simulink model "Tiefpass"  (R2023b)
settings: Solver=VariableStepAuto  StartTime=0.0  StopTime=1  RelTol=1e-3
settings Model: Creator=Adrian  LastModifiedBy=Adrian

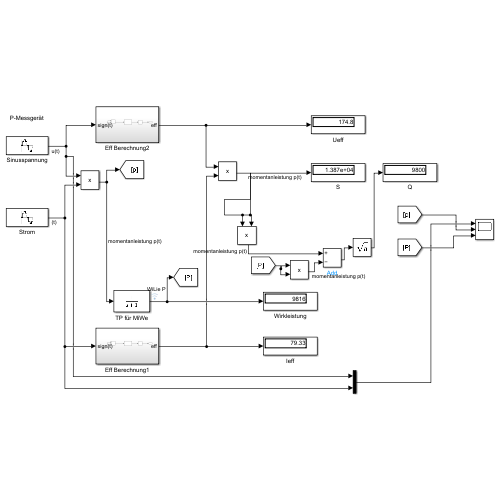
[thumbnail: Simulink's stored preview of the top-level diagram]
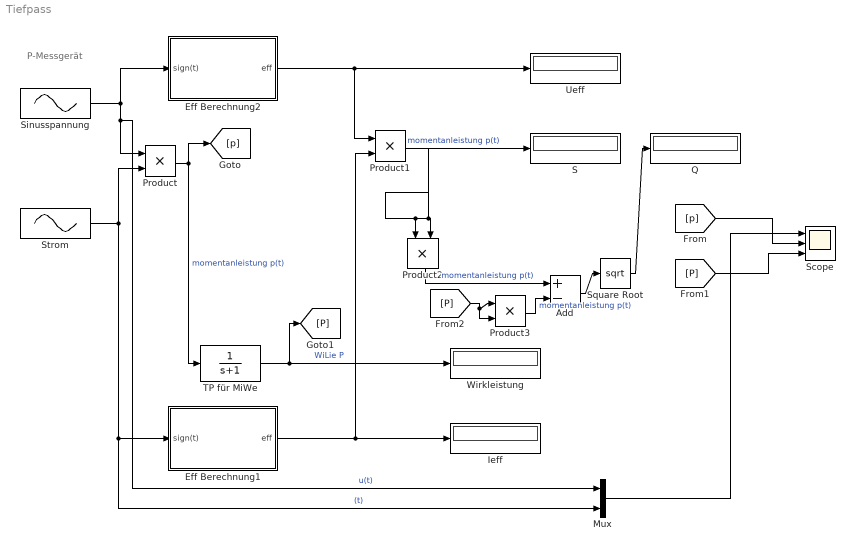
== system Tiefpass ==
  note: P-Messgerät
  Add : Sum  Inputs=+-
  Eff Berechnung1 : Subsystem
  Eff Berechnung2 : Subsystem
  Ieff : Display
  Mux : Mux  Inputs=2
  Product{,1..3} (4 alike) : Product
  Q : Display
  S : Display
  Scope : Scope  NumInputPorts=3
  Sinusspannung : Sin  Amplitude=311  Frequency=50*2*pi  SampleTime=0.1e-3
  Square Root : Sqrt
  Strom : Sin  Amplitude=141  Frequency=50*2*pi  Phase=-45*pi/180  SampleTime=0.1e-3
  TP für MiWe : TransferFcn  Denominator=[1 1]
  Ueff : Display
  Wirkleistung : Display
  wires:
  Strom/1 -> Mux/2, Eff Berechnung1/1(sign(t)), Product/2  "(t)"
  Sinusspannung/1 -> Mux/1, Product/1, Eff Berechnung2/1(sign(t))  "u(t)"
  Mux/1 -> Scope/1
  Product/1 -> [p], TP für MiWe/1  "momentanleistung p(t)"
  TP für MiWe/1 -> [P], Wirkleistung/1  "WiLie P"
  Eff Berechnung2/1(eff) -> Ueff/1, Product1/1
  Eff Berechnung1/1(eff) -> Product1/2, Ieff/1
  [p] -> Scope/2
  [P] -> Scope/3
  Product1/1 -> Product2/1, S/1, Product2/2  "momentanleistung p(t)"
  [P] -> Product3/2, Product3/1
  Product2/1 -> Add/1  "momentanleistung p(t)"
  Product3/1 -> Add/2  "momentanleistung p(t)"
  Add/1 -> Square Root/1
  Square Root/1 -> Q/1

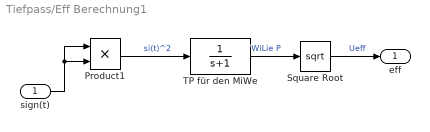
== system Tiefpass/Eff Berechnung1 ==
  sign(t) : Inport
  Product1 : Product
  Square Root : Sqrt
  TP für den MiWe : TransferFcn  Denominator=[1 1]
  eff : Outport
  wires:
  Product1/1 -> TP für den MiWe/1  "si(t)^2"
  sign(t)/1 -> Product1/1, Product1/2
  TP für den MiWe/1 -> Square Root/1  "WiLie P"
  Square Root/1 -> eff/1  "Ueff"

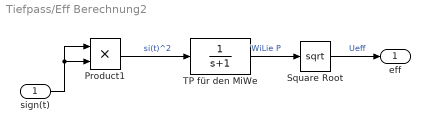
== system Tiefpass/Eff Berechnung2 ==
  sign(t) : Inport
  Product1 : Product
  Square Root : Sqrt
  TP für den MiWe : TransferFcn  Denominator=[1 1]
  eff : Outport
  wires:
  Product1/1 -> TP für den MiWe/1  "si(t)^2"
  sign(t)/1 -> Product1/1, Product1/2
  TP für den MiWe/1 -> Square Root/1  "WiLie P"
  Square Root/1 -> eff/1  "Ueff"
